simulink library "csu_mup_measurement_update_lib"  (R2014b)
settings: Solver=ode45  SolverMode=SingleTasking  StartTime=0.0  StopTime=10.0  RelTol=1e-3
values from neighbouring files (symbols this model uses):
  mup_columns = [1 : kfl_n_state]    [csu_mup_measurement_update_init.m]
  mup_identity = eye(kfl_n_state)    [csu_mup_measurement_update_init.m]
  mup_inovation_limits = [ 6000 0.5 0.5 0.1 0.1 0.1]    [csu_mup_measurement_update_init.m]
undefined symbols (not defined in the file or in its folder): kfl_n_state
libraries: util_info_lib x1
settings Model: Creator=escrane  LastModifiedBy=jimkaidy

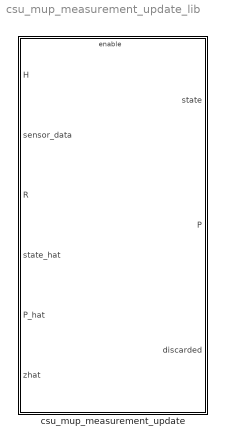
== system csu_mup_measurement_update_lib ==
  csu_mup_measurement_update : Subsystem

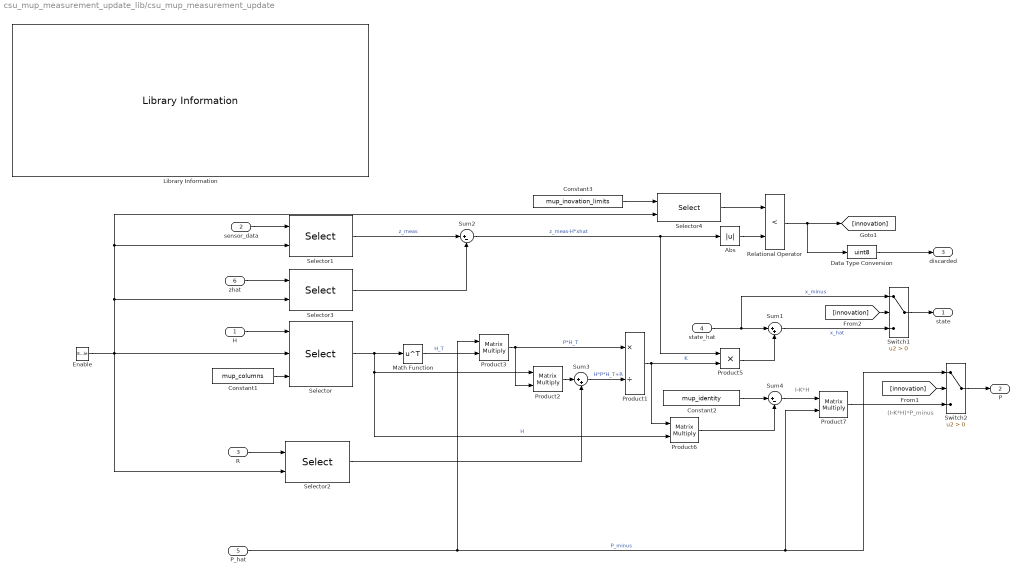
== system csu_mup_measurement_update_lib/csu_mup_measurement_update ==
  note: (I-K*H)*P_minus
  note: I-K*H
  H : Inport
  sensor_data : Inport  Port=2
  R : Inport  Port=3
  state_hat : Inport  Port=4
  P_hat : Inport  Port=5
  zhat : Inport  Port=6
  Enable : EnablePort  ShowOutputPort=on
  Abs : Abs
  Constant1 : Constant  Value=mup_columns  VectorParams1D=off
  Constant2 : Constant  Value=mup_identity
  Constant3 : Constant  Value=mup_inovation_limits  VectorParams1D=off
  Data Type Conversion : DataTypeConversion  OutDataTypeStr=uint8
  Library Information : util_info_lib/Library Information  owner='NONE'
  Math Function : Math  Operator=transpose  SaturateOnIntegerOverflow=on
  Product1 : Product  Inputs=*/  RndMeth=Zero
  Product{2..3,6..7} (4 alike) : Product  Multiplication=Matrix(*)  RndMeth=Zero
  Product5 : Product  RndMeth=Zero
  Relational Operator : RelationalOperator  Operator=<  OutDataTypeStr=boolean
  Selector : Selector  NumberOfDimensions=2  InputPortWidth=3  IndexOptions=Index vector (port),Index vector (port)  Indices=[1 3],1  OutputSizes=1,1
  Selector{1..4} (4 alike) : Selector  InputPortWidth=kfl_n_meas  IndexOptions=Index vector (port)  Indices=[1 3]
  Sum1 : Sum  Inputs=|++
  Sum2 : Sum  Inputs=|+-
  Sum3 : Sum  Inputs=|++
  Sum4 : Sum  Inputs=|+-
  Switch1 : Switch  Criteria=u2 > Threshold
  Switch2 : Switch  Criteria=u2 > Threshold
  state : Outport  OutDataTypeStr=double  InitialOutput=zeros(kfl_n_state,1)
  P : Outport  Port=2  OutDataTypeStr=double  InitialOutput=zeros(kfl_n_state, kfl_n_state)
  discarded : Outport  Port=3  OutDataTypeStr=uint8  OutputWhenDisabled=reset  InitialOutput=uint8(0)
  wires:
  Data Type Conversion/1 -> discarded/1
  Relational Operator/1 -> [innovation], Data Type Conversion/1
  Abs/1 -> Relational Operator/2
  Constant3/1 -> Selector4/1
  Selector4/1 -> Relational Operator/1
  Switch2/1 -> P/1
  Product7/1 -> Switch2/3
  [innovation] -> Switch2/2
  Switch1/1 -> state/1
  Sum1/1 -> Switch1/3  "x_hat"
  [innovation] -> Switch1/2
  Selector3/1 -> Sum2/2
  zhat/1 -> Selector3/1
  P_hat/1 -> Product3/1, Switch2/1, Product7/2  "P_minus"
  Sum4/1 -> Product7/1
  Product6/1 -> Sum4/2
  Constant2/1 -> Sum4/1
  Sum2/1 -> Abs/1, Product5/1  "z_meas-H*xhat"
  Product1/1 -> Product5/2, Product6/1  "K"
  Selector1/1 -> Sum2/1  "z_meas"
  sensor_data/1 -> Selector1/1
  Sum3/1 -> Product1/2  "H*P*H_T+R"
  Selector2/1 -> Sum3/2
  Product2/1 -> Sum3/1
  Product3/1 -> Product1/1, Product2/2  "P*H_T"
  Math Function/1 -> Product3/2  "H_T"
  state_hat/1 -> Sum1/1, Switch1/1  "x_minus"
  Selector/1 -> Product6/2, Product2/1, Math Function/1  "H"
  Enable/1 -> Selector3/2, Selector1/2, Selector4/2, Selector/2, Selector2/2
  R/1 -> Selector2/1
  H/1 -> Selector/1
  Constant1/1 -> Selector/3
  Product5/1 -> Sum1/2
